simulink model "ALC4"  (R2021b)
settings: Solver=VariableStepAuto  StartTime=0.0  StopTime=10.0  RelTol=1e-3
settings Model: Creator=wangm32  LastModifiedBy=wangm32

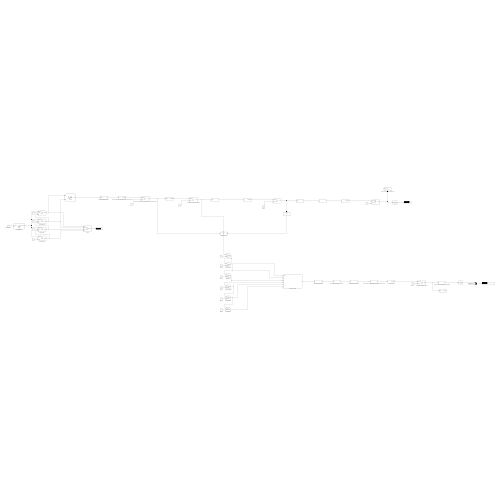
[thumbnail: Simulink's stored preview of the top-level diagram]
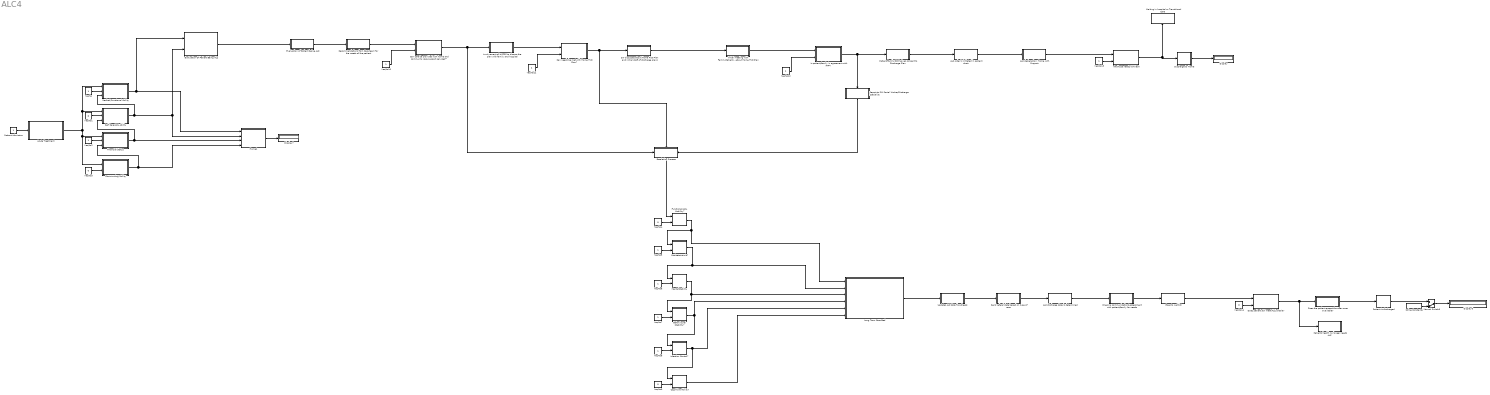
== system ALC4 ==
  ALC designation: Home with Support : Subsystem
  ALC discharge date is determined : Subsystem
  ALC order is initiated in patient chart : Subsystem
  Acute Treatment : Stateflow chart  TreatAsAtomicUnit=on
      settings: PortSchema="{\"entries\":[{\"content\":{\"sides\":[{\"content\":{\"connectorIds\":[\"In1\"]},\"type\":\"ConnectorPlacement.EquallySpacedRectSide\",\"uuid\":\"0242e5ac-2dba-41ea-8846-78efbd6bc89e\"},{\"content\":{\"connectorIds\":[\"Out1\"],\"side\":\"RIGHT\"},\"type\":\"ConnectorPlacement.EquallySpacedRectSide\",\"uuid\":\"e1122967-b177-4f42-90a1-fbb2908b74cb\"},{\"content\":{\"connectorIds\":[],\"side\":\"TOP\"},\"type\":\"ConnectorPlacement.EquallySpacedRectSide\",\"uuid\":\"f691757a-3ef2-4d8c-a42d-4ca76f7d4802\"},{\"content\":{\"connectorIds\":[\"In2\"],\"side\":\"BOTTOM\"},\"type\":\"ConnectorPlacement.EquallySpacedRectSide\",\"uuid\":\"5b499f63-ecd5-45be-9a9b-152b74a135c1\"}]},\"type\":\"ConnectorPlacement.EquallySpacedConnector\",\"uuid\":\"14c49482-40e8-45f5-ad45-681a46d0b3ed\"}],\"packageUris\":[\"http://schema.mathworks.com/mf0/Connector/R2020b\"],\"version\":\"1.0\"}"
  Are those needs fulfilled? : Stateflow chart  TreatAsAtomicUnit=on
      settings: PortSchema="{\"entries\":[{\"content\":{\"sides\":[{\"content\":{\"connectorIds\":[\"In1\",\"In2\"]},\"type\":\"ConnectorPlacement.EquallySpacedRectSide\",\"uuid\":\"6bdd9e00-5391-47d3-8f9d-9d8f069e16dc\"},{\"content\":{\"connectorIds\":[\"Out1\"],\"side\":\"RIGHT\"},\"type\":\"ConnectorPlacement.EquallySpacedRectSide\",\"uuid\":\"f5245c00-1436-4385-a45e-18909dc5d05a\"},{\"content\":{\"connectorIds\":[\"In3\"],\"side\":\"TOP\"},\"type\":\"ConnectorPlacement.EquallySpacedRectSide\",\"uuid\":\"337eeddb-d5e9-4089-85da-63e081b06c27\"}]},\"type\":\"ConnectorPlacement.EquallySpacedConnector\",\"uuid\":\"e179e3d5-aa42-4786-98a2-0c1e0c5c0d89\"}],\"packageUris\":[\"http://schema.mathworks.com/mf0/Connector/R2020b\"],\"version\":\"1.0\"}"
  "Behavioural Stability? " : Stateflow chart  TreatAsAtomicUnit=on
  Can care be provided with home and community care support services?* : Stateflow chart  TreatAsAtomicUnit=on
  Can needs be met with Home First Plan? : Stateflow chart  TreatAsAtomicUnit=on
  Cognitive Ability? : Stateflow chart  TreatAsAtomicUnit=on
  Communting Ability : Stateflow chart  TreatAsAtomicUnit=on
  Discharge to Home : Stateflow chart  TreatAsAtomicUnit=on
  Display : Display
  Display6 : Display
  Display7 : Display
  Does patient still meet ALC criteria? : Stateflow chart  TreatAsAtomicUnit=on
  Does the patient accept the offer once available? : Subsystem
  Escalation Process : Subsystem
      settings: PortSchema="{\"entries\":[{\"content\":{\"sides\":[{\"content\":{\"connectorIds\":[\"In1\"]},\"type\":\"ConnectorPlacement.EquallySpacedRectSide\",\"uuid\":\"6bdd9e00-5391-47d3-8f9d-9d8f069e16dc\"},{\"content\":{\"connectorIds\":[\"In3\"],\"side\":\"RIGHT\"},\"type\":\"ConnectorPlacement.EquallySpacedRectSide\",\"uuid\":\"f5245c00-1436-4385-a45e-18909dc5d05a\"},{\"content\":{\"connectorIds\":[\"In2\"],\"side\":\"TOP\"},\"type\":\"ConnectorPlacement.EquallySpacedRectSide\",\"uuid\":\"337eeddb-d5e9-4089-85da-63e081b06c27\"},{\"content\":{\"connectorIds\":[\"Out1\"],\"side\":\"BOTTOM\"},\"type\":\"ConnectorPlacement.EquallySpacedRectSide\",\"uuid\":\"2dffb6ac-bff8-4a73-b1c4-a44c996c4cd6\"}]},\"type\":\"ConnectorPlacement.EquallySpacedConnector\",\"uuid\":\"e179e3d5-aa42-4786-98a2-0c1e0c5c0d89\"}],\"packageUris\":[\"http://schema.mathworks.com/mf0/Connector/R2020b\"],\"version\":\"1.0\"}"
  Evaluation Of Patient Being ALC : Stateflow chart  TreatAsAtomicUnit=on
  Evaluation of Patient being ALC : Subsystem
  Financial Status : Stateflow chart  TreatAsAtomicUnit=on
  Functional/ADL Mobility? : Stateflow chart  TreatAsAtomicUnit=on
  Goes to waitlist : Subsystem
  Home1 : Stateflow chart  TreatAsAtomicUnit=on
  "Infection Control? " : Stateflow chart  TreatAsAtomicUnit=on
  Initial meeting with Family/Patient/Health Care Team about Home First Plan : Subsystem
  Involvement of HCCSS to discuss the plan with family and hospital : Subsystem
  Is patient/family in agreement with HFP? : Stateflow chart  TreatAsAtomicUnit=on
  Long Term Care Bed : Subsystem
  Manual Switch6 : ManualSwitch  CurrentSetting=0
  Medical/Functional Ability : Stateflow chart  TreatAsAtomicUnit=on
  "MentalStability " : Stateflow chart  TreatAsAtomicUnit=on
  Ongoing communication&assessment with patient/family for needs : Subsystem
  Patient Admission : Constant
  Patient is discharged : Stateflow chart  TreatAsAtomicUnit=on
  Patient/Family/SDM gives consent to Discharge Plan : Subsystem
  Patients health no longer needs ALC : Subsystem
  Recommendations from Care team for the needs of the patient : Subsystem
  Report to SW Social Worker/Discharge specialist : Subsystem
      settings: PortSchema="{\"entries\":[{\"content\":{\"sides\":[{\"content\":{\"connectorIds\":[]},\"type\":\"ConnectorPlacement.EquallySpacedRectSide\",\"uuid\":\"2efda515-0993-4186-88e6-75ed01c0ca4f\"},{\"content\":{\"connectorIds\":[],\"side\":\"RIGHT\"},\"type\":\"ConnectorPlacement.EquallySpacedRectSide\",\"uuid\":\"df20f571-132d-4593-9e22-0c1c06cb05bd\"},{\"content\":{\"connectorIds\":[\"In1\"],\"side\":\"TOP\"},\"type\":\"ConnectorPlacement.EquallySpacedRectSide\",\"uuid\":\"3e1d8c0a-53c7-420f-8f41-84478c44449b\"},{\"content\":{\"connectorIds\":[\"Out1\"],\"side\":\"BOTTOM\"},\"type\":\"ConnectorPlacement.EquallySpacedRectSide\",\"uuid\":\"6bf3d86e-aa45-459a-bcba-53e0327c35e7\"}]},\"type\":\"ConnectorPlacement.EquallySpacedConnector\",\"uuid\":\"974ce28f-d225-405a-a6db-52038ff460e7\"}],\"packageUris\":[\"http://schema.mathworks.com/mf0/Connector/R2020b\"],\"version\":\"1.0\"}"
  SW discusses about Home First Plan and initial draft of discharge plans : Subsystem
  Self Care/ADL Ability : Stateflow chart  TreatAsAtomicUnit=on
  Send referal date based on type of care : Subsystem
  Socioeconomic? : Stateflow chart  TreatAsAtomicUnit=on
  String Constant6 : StringConstant  String="\"Deactived\""
  Updates ALC data flowsheets : Subsystem
  Waiting in hospital or Transitional Care : Subsystem
      settings: PortSchema="{\"entries\":[{\"content\":{\"sides\":[{\"content\":{\"connectorIds\":[\"Out1\"]},\"type\":\"ConnectorPlacement.EquallySpacedRectSide\",\"uuid\":\"2efda515-0993-4186-88e6-75ed01c0ca4f\"},{\"content\":{\"connectorIds\":[],\"side\":\"RIGHT\"},\"type\":\"ConnectorPlacement.EquallySpacedRectSide\",\"uuid\":\"df20f571-132d-4593-9e22-0c1c06cb05bd\"},{\"content\":{\"connectorIds\":[],\"side\":\"TOP\"},\"type\":\"ConnectorPlacement.EquallySpacedRectSide\",\"uuid\":\"3e1d8c0a-53c7-420f-8f41-84478c44449b\"},{\"content\":{\"connectorIds\":[\"In1\"],\"side\":\"BOTTOM\"},\"type\":\"ConnectorPlacement.EquallySpacedRectSide\",\"uuid\":\"95f2a6b8-43c0-48c5-ae07-276b7c410744\"}]},\"type\":\"ConnectorPlacement.EquallySpacedConnector\",\"uuid\":\"974ce28f-d225-405a-a6db-52038ff460e7\"}],\"packageUris\":[\"http://schema.mathworks.com/mf0/Connector/R2020b\"],\"version\":\"1.0\"}"
  Yes/No{,2,5..8,10..13} (10 alike) : Constant
  Yes/No{1,3..4,9,14} (5 alike) : Constant  Value=0
  wires:
  Yes/No9/1 -> Cognitive Ability?/2(choice)
  Functional/ADL Mobility?/1(output) -> Long Term Care Bed/1(output), Socioeconomic?/1(Pre)
  Communting Ability/1(output) -> Home1/4(CA), Financial Status/3(CA)
  Yes/No7/1 -> "Behavioural Stability? "/2(choice)
  "Infection Control? "/1(output) -> Long Term Care Bed/5(In5), Cognitive Ability?/1(Pre)
  "MentalStability "/1(output) -> Long Term Care Bed/3(In4), "Behavioural Stability? "/1(Pre)
  Yes/No4/1 -> Functional/ADL Mobility?/2(choice)
  Yes/No8/1 -> "Infection Control? "/2(choice)
  Yes/No6/1 -> "MentalStability "/2(choice)
  Patient Admission/1 -> Acute Treatment/1(admission)
  Cognitive Ability?/1(output) -> Long Term Care Bed/6(In6)
  "Behavioural Stability? "/1(output) -> Long Term Care Bed/4(In3), "Infection Control? "/1(Pre)
  Financial Status/1(output) -> Home1/3(FS), Self Care/ADL Ability/3(FS)
  Yes/No3/1 -> Communting Ability/2(choice)
  Yes/No5/1 -> Socioeconomic?/2(choice)
  Medical/Functional Ability/1(output) -> Home1/1(MA), Evaluation Of Patient Being ALC/1(MA)
  Evaluation Of Patient Being ALC/1(output) -> Evaluation of Patient being ALC/1(output)
  Yes/No2/1 -> Financial Status/2(choice)
  Self Care/ADL Ability/1(output) -> Medical/Functional Ability/3(SA), Home1/2(SCADL), Evaluation Of Patient Being ALC/2(SA)
  Yes/No/1 -> Medical/Functional Ability/2(choice)
  Yes/No1/1 -> Self Care/ADL Ability/2(choice)
  Acute Treatment/1(assesment) -> Communting Ability/1(assesment), Financial Status/1(assesment), Self Care/ADL Ability/1(assesment), Medical/Functional Ability/1(assesment)
  Socioeconomic?/1(output) -> Long Term Care Bed/2(In2), "MentalStability "/1(Pre)
  Evaluation of Patient being ALC/1(Out1) -> Recommendations from Care team for the needs of the patient/1(In1)
  Yes/No10/1 -> Can care be provided with home and community care support services?*/2(choice)
  Recommendations from Care team for the needs of the patient/1(assesment) -> Can care be provided with home and community care support services?*/1(assesment)
  Can care be provided with home and community care support services?*/1(output) -> Escalation Process/1(In3), Involvement of HCCSS to discuss the plan with family and hospital/1(output)
  Yes/No11/1 -> Can needs be met with Home First Plan?/2(choice)
  Involvement of HCCSS to discuss the plan with family and hospital/1(assesment) -> Can needs be met with Home First Plan?/1(assesment)
  Can needs be met with Home First Plan?/1(output) -> SW discusses about Home First Plan and initial draft of discharge plans/1(output), Escalation Process/2(output)
  SW discusses about Home First Plan and initial draft of discharge plans/1(Out1) -> Initial meeting with Family/Patient/Health Care Team about Home First Plan/1(In1)
  Yes/No12/1 -> Is patient/family in agreement with HFP?/2(choice)
  Initial meeting with Family/Patient/Health Care Team about Home First Plan/1(assesment) -> Is patient/family in agreement with HFP?/1(assesment)
  Is patient/family in agreement with HFP?/1(output) -> Report to SW Social Worker/Discharge specialist/1(output), Patient/Family/SDM gives consent to Discharge Plan/1(output)
  Patient/Family/SDM gives consent to Discharge Plan/1(Out1) -> ALC order is initiated in patient chart/1(In1)
  ALC order is initiated in patient chart/1(Out1) -> ALC designation: Home with Support/1(In1)
  Yes/No13/1 -> Are those needs fulfilled?/2(choice)
  ALC designation: Home with Support/1(assesment) -> Are those needs fulfilled?/1(assesment)
  Discharge to Home/1(output) -> Display/1
  Report to SW Social Worker/Discharge specialist/1(Out1) -> Escalation Process/3(In1)
  Escalation Process/1(ALC) -> Functional/ADL Mobility?/1(ALC)
  Long Term Care Bed/1(Out1) -> Updates ALC data flowsheets/1(In1)
  Updates ALC data flowsheets/1(Out1) -> Send referal date based on type of care/1(In1)
  Send referal date based on type of care/1(Out1) -> ALC discharge date is determined/1(In1)
  ALC discharge date is determined/1(Out1) -> Ongoing communication&assessment with patient/family for needs/1(In1)
  Ongoing communication&assessment with patient/family for needs/1(Out1) -> Goes to waitlist/1(In1)
  Yes/No14/1 -> Does patient still meet ALC criteria?/2(choice)
  Does patient still meet ALC criteria?/1(output) -> Patients health no longer needs ALC/1(output), Does the patient accept the offer once available?/1(In1)
  Goes to waitlist/1(assesment) -> Does patient still meet ALC criteria?/1(assesment)
  Manual Switch6/1 -> Display6/1
  String Constant6/1 -> Manual Switch6/2
  Patient is discharged/1(output) -> Manual Switch6/1
  Does the patient accept the offer once available?/1(ALC) -> Patient is discharged/1(ALC)
  Home1/1(output) -> Display7/1
  Are those needs fulfilled?/1(output) -> Discharge to Home/1(ALC), Waiting in hospital or Transitional Care/1(output)

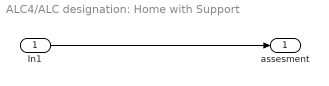
== system ALC4/ALC designation: Home with Support ==
  In1 : Inport
  assesment : Outport
  wires:
  In1/1 -> assesment/1

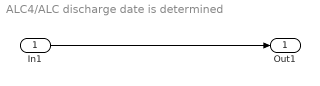
== system ALC4/ALC discharge date is determined ==
  In1 : Inport
  Out1 : Outport
  wires:
  In1/1 -> Out1/1

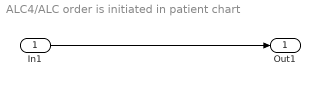
== system ALC4/ALC order is initiated in patient chart ==
  In1 : Inport
  Out1 : Outport
  wires:
  In1/1 -> Out1/1

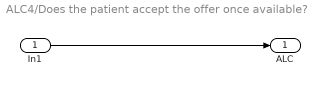
== system ALC4/Does the patient accept the offer once available? ==
  In1 : Inport
  ALC : Outport
  wires:
  In1/1 -> ALC/1

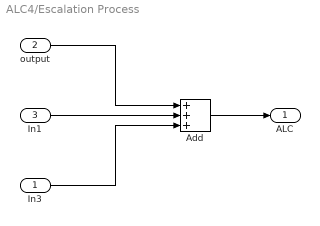
== system ALC4/Escalation Process ==
  In3 : Inport
  output : Inport  Port=2
  In1 : Inport  Port=3
  Add : Sum  Inputs=+++
  ALC : Outport
  wires:
  In1/1 -> Add/2
  output/1 -> Add/1
  In3/1 -> Add/3
  Add/1 -> ALC/1

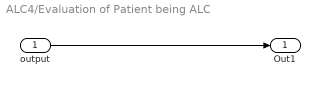
== system ALC4/Evaluation of Patient being ALC ==
  output : Inport
  Out1 : Outport
  wires:
  output/1 -> Out1/1

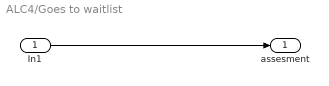
== system ALC4/Goes to waitlist ==
  In1 : Inport
  assesment : Outport
  wires:
  In1/1 -> assesment/1

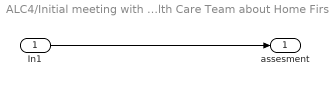
== system ALC4/Initial meeting with Family//Patient//Health Care Team about Home First Plan ==
  In1 : Inport
  assesment : Outport
  wires:
  In1/1 -> assesment/1

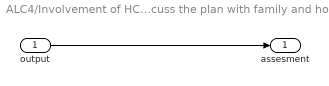
== system ALC4/Involvement of HCCSS to discuss the plan with family and hospital ==
  output : Inport
  assesment : Outport
  wires:
  output/1 -> assesment/1

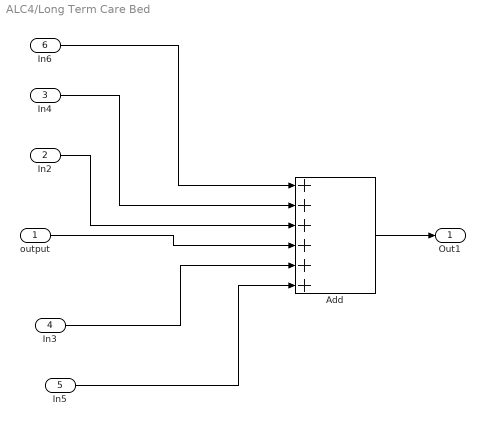
== system ALC4/Long Term Care Bed ==
  output : Inport
  In2 : Inport  Port=2
  In4 : Inport  Port=3
  In3 : Inport  Port=4
  In5 : Inport  Port=5
  In6 : Inport  Port=6
  Add : Sum  Inputs=++++++
  Out1 : Outport
  wires:
  Add/1 -> Out1/1
  In6/1 -> Add/1
  In4/1 -> Add/2
  In2/1 -> Add/3
  output/1 -> Add/4
  In3/1 -> Add/5
  In5/1 -> Add/6

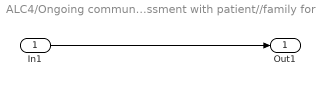
== system ALC4/Ongoing communication&assessment with patient//family for needs ==
  In1 : Inport
  Out1 : Outport
  wires:
  In1/1 -> Out1/1

== system ALC4/Patient//Family//SDM gives consent to Discharge Plan ==
  output : Inport
  Out1 : Outport
  wires:
  output/1 -> Out1/1

== system ALC4/Patients health no longer needs ALC ==
  output : Inport
  needcare : Outport
  wires:
  output/1 -> needcare/1

== system ALC4/Recommendations from Care team for the needs of the patient ==
  In1 : Inport
  assesment : Outport
  wires:
  In1/1 -> assesment/1

== system ALC4/Report to SW Social Worker//Discharge specialist ==
  output : Inport
  Out1 : Outport
  wires:
  output/1 -> Out1/1

== system ALC4/SW discusses about Home First Plan and initial draft of discharge plans ==
  output : Inport
  Out1 : Outport
  wires:
  output/1 -> Out1/1

== system ALC4/Send referal date based on type of care ==
  In1 : Inport
  Out1 : Outport
  wires:
  In1/1 -> Out1/1

== system ALC4/Updates ALC data flowsheets ==
  In1 : Inport
  Out1 : Outport
  wires:
  In1/1 -> Out1/1

== system ALC4/Waiting in hospital or Transitional Care ==
  output : Inport
  waiting : Outport
  wires:
  output/1 -> waiting/1

== stateflow chart ALC4/Functional//ADL Mobility? ==
  state ALC
  state FunctionalADLMobility
    entry:
  state yes
    entry:
    output=1;
  state no
    entry:
    output=0;
  (default) -> ALC
  ALC -> FunctionalADLMobility : [ALC==1]
  FunctionalADLMobility -> yes [order 1] : [choice==1]
  FunctionalADLMobility -> no [order 2]
  data: ALC input; choice input; output output

== stateflow chart ALC4/Socioeconomic? ==
  state ALC
  state Socioeconomic
    entry:
  state yes
    entry:
    output=1;
  state no
    entry:
    output=0;
  (default) -> ALC
  ALC -> Socioeconomic : [Pre==1]
  Socioeconomic -> yes [order 1] : [choice==1]
  Socioeconomic -> no [order 2]
  data: Pre input; choice input; output output

== stateflow chart ALC4/MentalStability  ==
  state ALC
  state MentalStability
    entry:
  state yes
    entry:
    output=1;
  state no
    entry:
    output=0;
  (default) -> ALC
  ALC -> MentalStability : [Pre==1]
  MentalStability -> yes [order 1] : [choice==1]
  MentalStability -> no [order 2]
  data: Pre input; choice input; output output

== stateflow chart ALC4/Behavioural Stability?  ==
  state ALC
  state BehaviouralStability
    entry:
  state yes
    entry:
    output=1;
  state no
    entry:
    output=0;
  (default) -> ALC
  ALC -> BehaviouralStability : [Pre==1]
  BehaviouralStability -> yes [order 1] : [choice==1]
  BehaviouralStability -> no [order 2]
  data: Pre input; choice input; output output

== stateflow chart ALC4/Infection Control?  ==
  state ALC
  state InfectionControl
    entry:
  state yes
    entry:
    output=1;
  state no
    entry:
    output=0;
  (default) -> ALC
  ALC -> InfectionControl : [Pre==1]
  InfectionControl -> yes [order 1] : [choice==1]
  InfectionControl -> no [order 2]
  data: Pre input; choice input; output output

== stateflow chart ALC4/Medical//Functional Ability ==
  state MFAbilityActived
    entry:
  state Assesment
  state yes
    output=1;
  state no
    output=0;
  (default) -> Assesment
  Assesment -> MFAbilityActived : [assesment==1||SA==0]
  MFAbilityActived -> yes [order 1] : [choice==1]
  MFAbilityActived -> no [order 2] : [choice==0]
  data: assesment input; choice input; output output; SA input

== stateflow chart ALC4/Cognitive Ability? ==
  state ALC
  state ADL
    entry:
  state yes
    entry:
    output=1;
  state no
    entry:
    output=0;
  (default) -> ALC
  ALC -> ADL : [Pre==1]
  ADL -> yes [order 1] : [choice==1]
  ADL -> no [order 2]
  data: Pre input; choice input; output output

== stateflow chart ALC4/Does patient still meet ALC criteria? ==
  state ALCCriterrica
    entry:
  state Assesment
  state yes
    output=1;
  state no
    output=0;
  (default) -> Assesment
  Assesment -> ALCCriterrica : [assesment==1]
  ALCCriterrica -> yes [order 1] : [choice==1]
  ALCCriterrica -> no [order 2] : [choice==0]
  data: assesment input; choice input; output output

== stateflow chart ALC4/Patient is discharged ==
  state Fcn
  state Result
    output="Patient is discharged successfully"
  (default) -> Fcn
  Fcn -> Result : [ALC==1]
  data: ALC input; output output

== stateflow chart ALC4/Can care be provided with home and community care support services?* ==
  state PSW_equipment_needs
    entry:
  state Assesment
  state yes
    output=1;
  state no
    output=0;
  (default) -> Assesment
  Assesment -> PSW_equipment_needs : [assesment==1]
  PSW_equipment_needs -> yes [order 1] : [choice==1]
  PSW_equipment_needs -> no [order 2] : [choice==0]
  data: assesment input; choice input; output output

== stateflow chart ALC4/Can needs be met with Home First Plan? ==
  state Home_First_Plan
    entry:
  state Assesment
  state yes
    output=1;
  state no
    output=0;
  (default) -> Assesment
  Assesment -> Home_First_Plan : [assesment==1]
  Home_First_Plan -> yes [order 1] : [choice==1]
  Home_First_Plan -> no [order 2] : [choice==0]
  data: assesment input; choice input; output output

== stateflow chart ALC4/Is patient//family in agreement with HFP? ==
  state HFP
    entry:
  state Assesment
  state yes
    output=1;
  state no
    output=0;
  (default) -> Assesment
  Assesment -> HFP : [assesment==1]
  HFP -> yes [order 1] : [choice==1]
  HFP -> no [order 2] : [choice==0]
  data: assesment input; choice input; output output

== stateflow chart ALC4/Are those needs fulfilled? ==
  state fulfilled_needs
    entry:
  state Assesment
  state yes
    output=1;
  state waiting
  state no
    output=0;
  (default) -> Assesment
  Assesment -> fulfilled_needs [order 1] : [assesment==1]
  fulfilled_needs -> yes [order 1] : [choice==1]
  Assesment -> waiting [order 2] : [waiting==1]
  fulfilled_needs -> no [order 2] : [choice==0]
  data: assesment input; choice input; output output; waiting input

== stateflow chart ALC4/Discharge to Home ==
  state Fcn
  state Result
    output="Home"
  (default) -> Fcn
  Fcn -> Result : [ALC==1]
  data: ALC input; output output

== stateflow chart ALC4/Self Care//ADL Ability ==
  state SCADLAbilityActived
    entry:
  state Assesment
  state yes
    output=1;
  state no
    output=0;
  (default) -> Assesment
  Assesment -> SCADLAbilityActived : [assesment==1||FS==0]
  SCADLAbilityActived -> yes [order 1] : [choice==1]
  SCADLAbilityActived -> no [order 2] : [choice==0]
  data: assesment input; choice input; output output; FS input

== stateflow chart ALC4/Acute Treatment ==
  state Medical_Condition
  state Medical_Assesment_
    entry:
    assesment=1;
  state Medical_Asses
    entry:
    assesment=1;
  (default) -> Medical_Condition
  Medical_Condition -> Medical_Assesment_ [order 1] : [admission==1]
  Medical_Condition -> Medical_Asses [order 2] : [needcare==1]
  data: admission input; assesment output; needcare input

== stateflow chart ALC4/Financial Status ==
  state FSActived
    entry:
  state Assesment
  state yes
    output=1;
  state no
    output=0;
  (default) -> Assesment
  Assesment -> FSActived : [assesment==1||CA==0]
  FSActived -> yes [order 1] : [choice==1]
  FSActived -> no [order 2] : [choice==0]
  data: assesment input; choice input; output output; CA input

== stateflow chart ALC4/Communting Ability ==
  state ComAbilityActived
    entry:
  state Assesment
  state yes
    output=1;
  state no
    output=0;
  (default) -> Assesment
  Assesment -> ComAbilityActived : [assesment==1]
  ComAbilityActived -> yes [order 1] : [choice==1]
  ComAbilityActived -> no [order 2] : [choice==0]
  data: assesment input; choice input; output output

== stateflow chart ALC4/Evaluation Of Patient Being ALC ==
  state EvaluationOfPatientBeingALC
  state output
    output=1;
  (default) -> EvaluationOfPatientBeingALC
  EvaluationOfPatientBeingALC -> output : [MA==0&&SA==0]
  data: MA input; SA input; output output

== stateflow chart ALC4/Home1 ==
  state Fcn
    input=MA+SCADL+FS+CA;
  state HomeActive
    entry:
    output="Home";
  state HomeDeActive
    entry:
    output="N/A";
  (default) -> Fcn
  Fcn -> HomeActive [order 1] : [input>3]
  Fcn -> HomeDeActive [order 2] : [input<3]
  data: MA input; SCADL input; FS input; CA input; output output; input local
